simulink model "Top"  (R2020b)
settings: Solver=VariableStepAuto  StartTime=0.0  StopTime=10.0  RelTol=1e-3
libraries: Bibavion x6
settings Model: Creator=Nicolas  LastModifiedBy=Nicolas

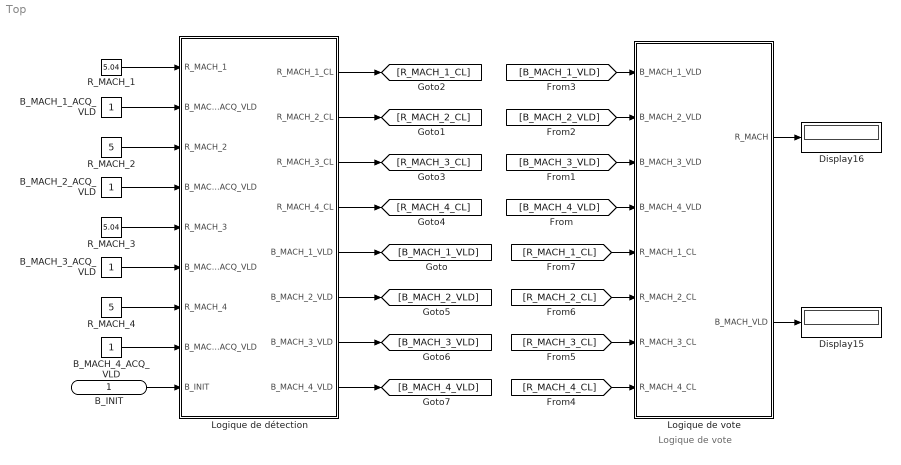
== system Top ==
  note: Logique de vote
  B_INIT : Inport  OutDataTypeStr=boolean
  B_MACH_1_ACQ_VLD : Constant  OutDataTypeStr=boolean
  B_MACH_2_ACQ_VLD : Constant  OutDataTypeStr=boolean
  B_MACH_3_ACQ_VLD : Constant  OutDataTypeStr=boolean
  B_MACH_4_ACQ_VLD : Constant  OutDataTypeStr=boolean
  Display15 : Display
  Display16 : Display
  Logique de détection : Subsystem
  Logique de vote : Subsystem
  R_MACH_1 : Constant  Value=5.04  OutDataTypeStr=single
  R_MACH_2 : Constant  Value=5  OutDataTypeStr=single
  R_MACH_3 : Constant  Value=5.04  OutDataTypeStr=single
  R_MACH_4 : Constant  Value=5  OutDataTypeStr=single
  wires:
  [B_MACH_4_VLD] -> Logique de vote/4(B_MACH_4_VLD)
  [R_MACH_1_CL] -> Logique de vote/5(R_MACH_1_CL)
  Logique de détection/4(R_MACH_4_CL) -> [R_MACH_4_CL]
  R_MACH_1/1 -> Logique de détection/1(R_MACH_1)
  B_MACH_3_ACQ_VLD/1 -> Logique de détection/6(B_MACH_3_ACQ_VLD)
  [R_MACH_4_CL] -> Logique de vote/8(R_MACH_4_CL)
  B_MACH_2_ACQ_VLD/1 -> Logique de détection/4(B_MACH_2_ACQ_VLD)
  Logique de détection/7(B_MACH_3_VLD) -> [B_MACH_3_VLD]
  R_MACH_3/1 -> Logique de détection/5(R_MACH_3)
  [B_MACH_3_VLD] -> Logique de vote/3(B_MACH_3_VLD)
  [R_MACH_3_CL] -> Logique de vote/7(R_MACH_3_CL)
  Logique de vote/2(B_MACH_VLD) -> Display15/1
  [B_MACH_2_VLD] -> Logique de vote/2(B_MACH_2_VLD)
  [R_MACH_2_CL] -> Logique de vote/6(R_MACH_2_CL)
  [B_MACH_1_VLD] -> Logique de vote/1(B_MACH_1_VLD)
  Logique de détection/1(R_MACH_1_CL) -> [R_MACH_1_CL]
  B_MACH_4_ACQ_VLD/1 -> Logique de détection/8(B_MACH_4_ACQ_VLD)
  B_MACH_1_ACQ_VLD/1 -> Logique de détection/2(B_MACH_1_ACQ_VLD)
  R_MACH_2/1 -> Logique de détection/3(R_MACH_2)
  Logique de détection/6(B_MACH_2_VLD) -> [B_MACH_2_VLD]
  Logique de détection/8(B_MACH_4_VLD) -> [B_MACH_4_VLD]
  Logique de détection/5(B_MACH_1_VLD) -> [B_MACH_1_VLD]
  Logique de vote/1(R_MACH) -> Display16/1
  R_MACH_4/1 -> Logique de détection/7(R_MACH_4)
  Logique de détection/2(R_MACH_2_CL) -> [R_MACH_2_CL]
  Logique de détection/3(R_MACH_3_CL) -> [R_MACH_3_CL]
  B_INIT/1 -> Logique de détection/9(B_INIT)

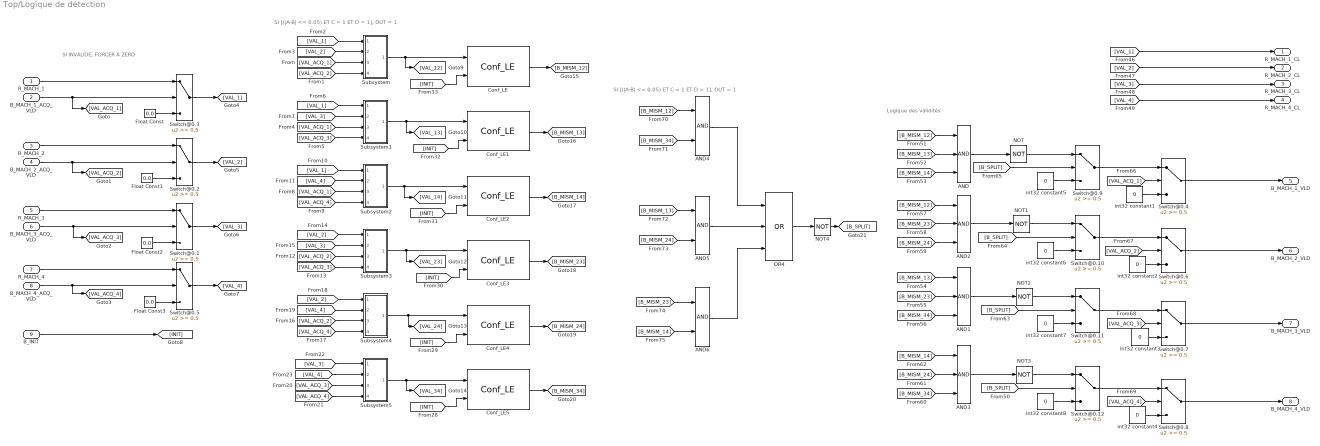
== system Top/Logique de détection ==
  note: SI [(|A-B| <= 0.05) ET C = 1 ET D = 1], OUT = 1
  note: SI INVALIDE, FORCER A ZERO
  note: Logique des validités
  note: SI [(|A-B| <= 0.05) ET C = 1 ET D = 1], OUT = 1
  R_MACH_1 : Inport
  B_MACH_1_ACQ_VLD : Inport  Port=2
  R_MACH_2 : Inport  Port=3
  B_MACH_2_ACQ_VLD : Inport  Port=4
  R_MACH_3 : Inport  Port=5
  B_MACH_3_ACQ_VLD : Inport  Port=6
  R_MACH_4 : Inport  Port=7
  B_MACH_4_ACQ_VLD : Inport  Port=8
  B_INIT : Inport  Port=9
  AND{,1..3} (4 alike) : Logic  Inputs=3  AllPortsSameDT=off  OutDataTypeStr=boolean
  AND4 : Logic  AllPortsSameDT=off  OutDataTypeStr=boolean
  AND5 : Logic  AllPortsSameDT=off  OutDataTypeStr=boolean
  AND6 : Logic  AllPortsSameDT=off  OutDataTypeStr=boolean
  Conf_LE{,1..5} (6 alike) : Bibavion/Logical/Conf_LE  time=2  init=0
      settings: SourceProductName=Bibavion P20
  Float Const{,1..3} (4 alike) : Constant  Value=0.0  OutDataTypeStr=single
  NOT{,1..4} (5 alike) : Logic  Operator=NOT  IconShape=distinctive  AllPortsSameDT=off  OutDataTypeStr=boolean
  OR4 : Logic  Operator=OR  Inputs=3  AllPortsSameDT=off  OutDataTypeStr=boolean
  Subsystem : Subsystem
  Subsystem1 : Subsystem
  Subsystem2 : Subsystem
  Subsystem3 : Subsystem
  Subsystem4 : Subsystem
  Subsystem5 : Subsystem
  Switch@0.{1..12} (12 alike) : Switch  Threshold=0.5
  int32 constant{1..8} (8 alike) : Constant  Value=0  OutDataTypeStr=int32  SampleTime=-1
  R_MACH_1_CL : Outport
  R_MACH_2_CL : Outport  Port=2
  R_MACH_3_CL : Outport  Port=3
  R_MACH_4_CL : Outport  Port=4
  B_MACH_1_VLD : Outport  Port=5
  B_MACH_2_VLD : Outport  Port=6
  B_MACH_3_VLD : Outport  Port=7
  B_MACH_4_VLD : Outport  Port=8
  wires:
  [VAL_ACQ_2] -> Subsystem4/3(In3)
  Float Const3/1 -> Switch@0.5/3
  [VAL_ACQ_2] -> Subsystem/4(In4)
  B_MACH_3_ACQ_VLD/1 -> [VAL_ACQ_3], Switch@0.1/2
  NOT1/1 -> Switch@0.10/1
  [B_MISM_23] -> AND1/2
  [VAL_ACQ_1] -> Subsystem2/3(In3)
  Switch@0.11/1 -> Switch@0.7/1
  AND4/1 -> OR4/1
  [VAL_4] -> Subsystem4/2(In2)
  [B_MISM_24] -> AND2/3
  Switch@0.3/1 -> [VAL_1]
  B_MACH_4_ACQ_VLD/1 -> Switch@0.5/2, [VAL_ACQ_4]
  B_MACH_1_ACQ_VLD/1 -> [VAL_ACQ_1], Switch@0.3/2
  Subsystem1/1(Out1) -> [VAL_13], Conf_LE1/1
  Switch@0.12/1 -> Switch@0.8/1
  [VAL_3] -> Subsystem1/2(In2)
  [VAL_ACQ_3] -> Subsystem1/4(In4)
  Float Const1/1 -> Switch@0.2/3
  [VAL_ACQ_1] -> Subsystem/3(In3)
  [VAL_1] -> Subsystem1/1(In1)
  Conf_LE3/1 -> [B_MISM_23]
  [VAL_2] -> Subsystem4/1(In1)
  [INIT] -> Conf_LE5/2
  Switch@0.2/1 -> [VAL_2]
  Conf_LE1/1 -> [B_MISM_13]
  Switch@0.8/1 -> B_MACH_4_VLD/1
  Subsystem5/1(Out1) -> [VAL_34], Conf_LE5/1
  B_MACH_2_ACQ_VLD/1 -> [VAL_ACQ_2], Switch@0.2/2
  [VAL_3] -> Subsystem3/2(In2)
  Switch@0.1/1 -> [VAL_3]
  [B_MISM_14] -> AND3/1
  [VAL_2] -> Subsystem3/1(In1)
  [VAL_2] -> Subsystem/2(In2)
  [VAL_ACQ_3] -> Switch@0.7/2
  Subsystem4/1(Out1) -> [VAL_24], Conf_LE4/1
  [VAL_1] -> R_MACH_1_CL/1
  [VAL_4] -> Subsystem2/2(In2)
  int32 constant3/1 -> Switch@0.7/3
  NOT4/1 -> [B_SPLIT]
  [VAL_4] -> Subsystem5/2(In2)
  Switch@0.7/1 -> B_MACH_3_VLD/1
  [VAL_ACQ_3] -> Subsystem5/3(In3)
  AND/1 -> NOT/1
  [VAL_ACQ_3] -> Subsystem3/4(In4)
  [B_MISM_24] -> AND5/2
  AND3/1 -> NOT3/1
  Subsystem2/1(Out1) -> [VAL_14], Conf_LE2/1
  [INIT] -> Conf_LE4/2
  [B_SPLIT] -> Switch@0.11/2
  [VAL_ACQ_4] -> Subsystem2/4(In4)
  R_MACH_1/1 -> Switch@0.3/1
  [INIT] -> Conf_LE2/2
  [VAL_ACQ_2] -> Subsystem3/3(In3)
  Float Const2/1 -> Switch@0.1/3
  Float Const/1 -> Switch@0.3/3
  [VAL_ACQ_4] -> Subsystem4/4(In4)
  [VAL_ACQ_2] -> Switch@0.6/2
  Subsystem/1(Out1) -> [VAL_12], Conf_LE/1
  Subsystem3/1(Out1) -> [VAL_23], Conf_LE3/1
  [VAL_1] -> Subsystem/1(In1)
  [VAL_2] -> R_MACH_2_CL/1
  Switch@0.10/1 -> Switch@0.6/1
  [INIT] -> Conf_LE/2
  [VAL_4] -> R_MACH_4_CL/1
  [VAL_ACQ_4] -> Subsystem5/4(In4)
  [B_MISM_13] -> AND5/1
  Switch@0.5/1 -> [VAL_4]
  AND6/1 -> OR4/3
  [VAL_1] -> Subsystem2/1(In1)
  [VAL_ACQ_1] -> Subsystem1/3(In3)
  NOT2/1 -> Switch@0.11/1
  [INIT] -> Conf_LE3/2
  [INIT] -> Conf_LE1/2
  [VAL_3] -> Subsystem5/1(In1)
  Conf_LE4/1 -> [B_MISM_24]
  int32 constant4/1 -> Switch@0.8/3
  [B_MISM_23] -> AND6/1
  Conf_LE/1 -> [B_MISM_12]
  [VAL_ACQ_4] -> Switch@0.8/2
  AND1/1 -> NOT2/1
  AND2/1 -> NOT1/1
  Conf_LE2/1 -> [B_MISM_14]
  [VAL_ACQ_1] -> Switch@0.4/2
  [B_MISM_14] -> AND/3
  [B_MISM_13] -> AND/2
  NOT/1 -> Switch@0.9/1
  [B_MISM_12] -> AND4/1
  [B_MISM_34] -> AND3/3
  Conf_LE5/1 -> [B_MISM_34]
  AND5/1 -> OR4/2
  int32 constant6/1 -> Switch@0.10/3
  [B_SPLIT] -> Switch@0.10/2
  int32 constant2/1 -> Switch@0.6/3
  [B_MISM_13] -> AND1/1
  [B_MISM_12] -> AND2/1
  [B_MISM_23] -> AND2/2
  Switch@0.4/1 -> B_MACH_1_VLD/1
  [B_MISM_12] -> AND/1
  OR4/1 -> NOT4/1
  int32 constant8/1 -> Switch@0.12/3
  [B_MISM_34] -> AND1/3
  [B_SPLIT] -> Switch@0.9/2
  [B_MISM_24] -> AND3/2
  NOT3/1 -> Switch@0.12/1
  int32 constant1/1 -> Switch@0.4/3
  [VAL_3] -> R_MACH_3_CL/1
  [B_MISM_14] -> AND6/2
  [B_MISM_34] -> AND4/2
  Switch@0.6/1 -> B_MACH_2_VLD/1
  int32 constant7/1 -> Switch@0.11/3
  Switch@0.9/1 -> Switch@0.4/1
  [B_SPLIT] -> Switch@0.12/2
  int32 constant5/1 -> Switch@0.9/3
  B_INIT/1 -> [INIT]
  R_MACH_2/1 -> Switch@0.2/1
  R_MACH_4/1 -> Switch@0.5/1
  R_MACH_3/1 -> Switch@0.1/1

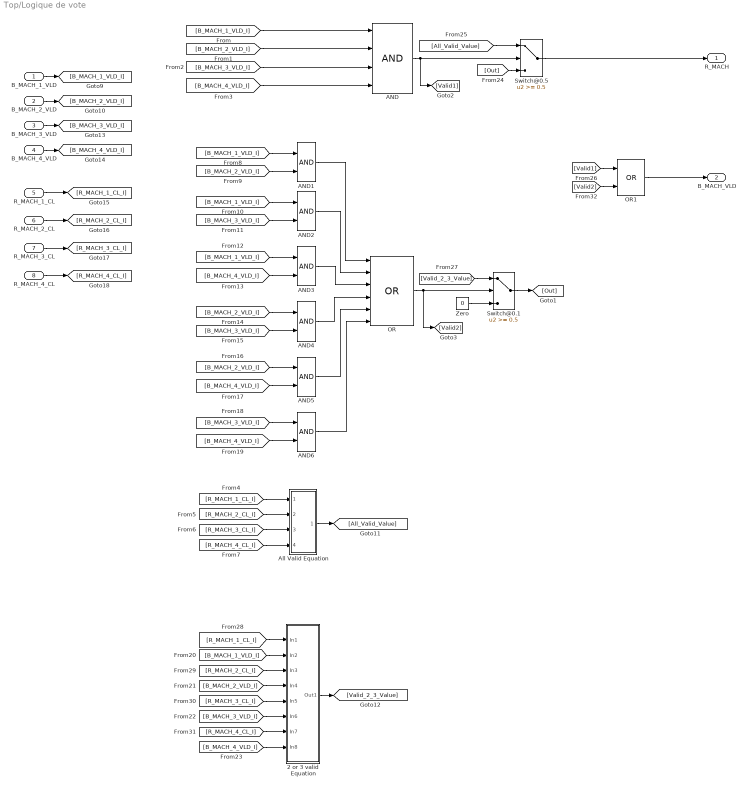
== system Top/Logique de vote ==
  B_MACH_1_VLD : Inport
  B_MACH_2_VLD : Inport  Port=2
  B_MACH_3_VLD : Inport  Port=3
  B_MACH_4_VLD : Inport  Port=4
  R_MACH_1_CL : Inport  Port=5
  R_MACH_2_CL : Inport  Port=6
  R_MACH_3_CL : Inport  Port=7
  R_MACH_4_CL : Inport  Port=8
  2 or 3 valid Equation : Subsystem
  AND : Logic  Inputs=4  IconShape=distinctive  AllPortsSameDT=off  OutDataTypeStr=boolean
  AND{1..6} (6 alike) : Logic  IconShape=distinctive  AllPortsSameDT=off  OutDataTypeStr=boolean
  All Valid Equation : Subsystem
  OR : Logic  Operator=OR  Inputs=6  IconShape=distinctive  AllPortsSameDT=off  OutDataTypeStr=boolean
  OR1 : Logic  Operator=OR  IconShape=distinctive  AllPortsSameDT=off  OutDataTypeStr=boolean
  Switch@0.1 : Switch  Threshold=0.5
  Switch@0.5 : Switch  Threshold=0.5
  Zero : Constant  Value=0  OutDataTypeStr=single
  R_MACH : Outport
  B_MACH_VLD : Outport  Port=2
  wires:
  [B_MACH_2_VLD_I] -> AND1/2
  B_MACH_3_VLD/1 -> [B_MACH_3_VLD_I]
  [B_MACH_2_VLD_I] -> AND/2
  [B_MACH_4_VLD_I] -> AND/4
  [B_MACH_1_VLD_I] -> AND/1
  R_MACH_2_CL/1 -> [R_MACH_2_CL_I]
  [B_MACH_3_VLD_I] -> AND2/2
  R_MACH_1_CL/1 -> [R_MACH_1_CL_I]
  [R_MACH_2_CL_I] -> All Valid Equation/2(In2)
  [B_MACH_4_VLD_I] -> AND3/2
  AND2/1 -> OR/2
  [B_MACH_2_VLD_I] -> AND5/1
  [B_MACH_1_VLD_I] -> AND2/1
  [B_MACH_3_VLD_I] -> AND4/2
  [B_MACH_3_VLD_I] -> AND/3
  R_MACH_4_CL/1 -> [R_MACH_4_CL_I]
  AND4/1 -> OR/4
  B_MACH_1_VLD/1 -> [B_MACH_1_VLD_I]
  AND/1 -> [Valid1], Switch@0.5/2
  [R_MACH_4_CL_I] -> 2 or 3 valid Equation/7(In7)
  [B_MACH_3_VLD_I] -> AND6/1
  [Valid_2_3_Value] -> Switch@0.1/1
  AND5/1 -> OR/5
  OR/1 -> [Valid2], Switch@0.1/2
  [B_MACH_1_VLD_I] -> AND1/1
  [B_MACH_1_VLD_I] -> AND3/1
  [B_MACH_3_VLD_I] -> 2 or 3 valid Equation/6(In6)
  B_MACH_4_VLD/1 -> [B_MACH_4_VLD_I]
  [B_MACH_4_VLD_I] -> AND6/2
  [R_MACH_1_CL_I] -> All Valid Equation/1(In1)
  2 or 3 valid Equation/1(Out1) -> [Valid_2_3_Value]
  [R_MACH_3_CL_I] -> All Valid Equation/3(In3)
  [B_MACH_4_VLD_I] -> AND5/2
  [B_MACH_1_VLD_I] -> 2 or 3 valid Equation/2(In2)
  [R_MACH_3_CL_I] -> 2 or 3 valid Equation/5(In5)
  [R_MACH_4_CL_I] -> All Valid Equation/4(In4)
  All Valid Equation/1(Out1) -> [All_Valid_Value]
  [All_Valid_Value] -> Switch@0.5/1
  AND3/1 -> OR/3
  [R_MACH_1_CL_I] -> 2 or 3 valid Equation/1(In1)
  [B_MACH_2_VLD_I] -> 2 or 3 valid Equation/4(In4)
  [R_MACH_2_CL_I] -> 2 or 3 valid Equation/3(In3)
  AND6/1 -> OR/6
  [B_MACH_4_VLD_I] -> 2 or 3 valid Equation/8(In8)
  [B_MACH_2_VLD_I] -> AND4/1
  AND1/1 -> OR/1
  Zero/1 -> Switch@0.1/3
  R_MACH_3_CL/1 -> [R_MACH_3_CL_I]
  Switch@0.5/1 -> R_MACH/1
  B_MACH_2_VLD/1 -> [B_MACH_2_VLD_I]
  Switch@0.1/1 -> [Out]
  [Out] -> Switch@0.5/3
  [Valid1] -> OR1/1
  [Valid2] -> OR1/2
  OR1/1 -> B_MACH_VLD/1

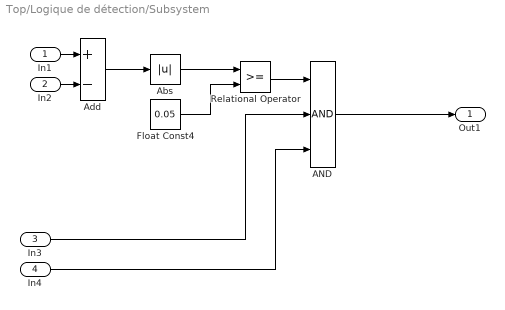
== system Top/Logique de détection/Subsystem ==
  In1 : Inport
  In2 : Inport  Port=2
  In3 : Inport  Port=3
  In4 : Inport  Port=4
  AND : Logic  Inputs=3  AllPortsSameDT=off  OutDataTypeStr=boolean
  Abs : Abs
  Add : Sum  Inputs=+-
  Float Const4 : Constant  Value=0.05  OutDataTypeStr=single
  Relational Operator : RelationalOperator  OutDataTypeStr=boolean  RndMeth=Nearest
  Out1 : Outport
  wires:
  In3/1 -> AND/2
  In4/1 -> AND/3
  Add/1 -> Abs/1
  Relational Operator/1 -> AND/1
  Abs/1 -> Relational Operator/1
  AND/1 -> Out1/1
  Float Const4/1 -> Relational Operator/2
  In2/1 -> Add/2
  In1/1 -> Add/1

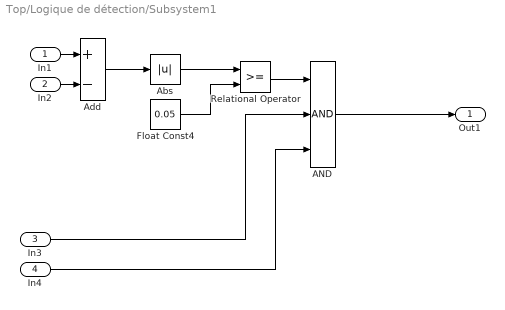
== system Top/Logique de détection/Subsystem1 ==
  In1 : Inport
  In2 : Inport  Port=2
  In3 : Inport  Port=3
  In4 : Inport  Port=4
  AND : Logic  Inputs=3  AllPortsSameDT=off  OutDataTypeStr=boolean
  Abs : Abs
  Add : Sum  Inputs=+-
  Float Const4 : Constant  Value=0.05  OutDataTypeStr=single
  Relational Operator : RelationalOperator  OutDataTypeStr=boolean  RndMeth=Nearest
  Out1 : Outport
  wires:
  In3/1 -> AND/2
  In4/1 -> AND/3
  Add/1 -> Abs/1
  Relational Operator/1 -> AND/1
  Abs/1 -> Relational Operator/1
  AND/1 -> Out1/1
  Float Const4/1 -> Relational Operator/2
  In2/1 -> Add/2
  In1/1 -> Add/1

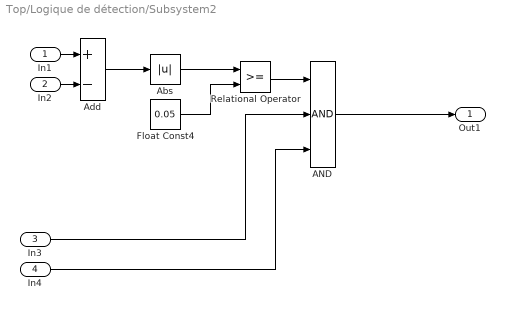
== system Top/Logique de détection/Subsystem2 ==
  In1 : Inport
  In2 : Inport  Port=2
  In3 : Inport  Port=3
  In4 : Inport  Port=4
  AND : Logic  Inputs=3  AllPortsSameDT=off  OutDataTypeStr=boolean
  Abs : Abs
  Add : Sum  Inputs=+-
  Float Const4 : Constant  Value=0.05  OutDataTypeStr=single
  Relational Operator : RelationalOperator  OutDataTypeStr=boolean  RndMeth=Nearest
  Out1 : Outport
  wires:
  In3/1 -> AND/2
  In4/1 -> AND/3
  Add/1 -> Abs/1
  Relational Operator/1 -> AND/1
  Abs/1 -> Relational Operator/1
  AND/1 -> Out1/1
  Float Const4/1 -> Relational Operator/2
  In2/1 -> Add/2
  In1/1 -> Add/1

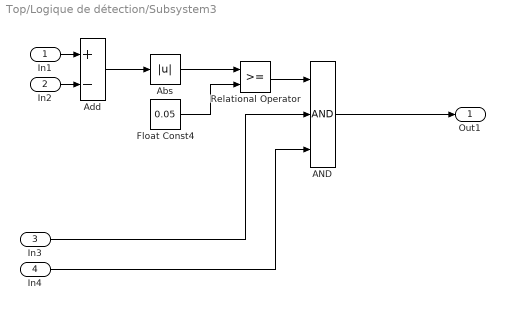
== system Top/Logique de détection/Subsystem3 ==
  In1 : Inport
  In2 : Inport  Port=2
  In3 : Inport  Port=3
  In4 : Inport  Port=4
  AND : Logic  Inputs=3  AllPortsSameDT=off  OutDataTypeStr=boolean
  Abs : Abs
  Add : Sum  Inputs=+-
  Float Const4 : Constant  Value=0.05  OutDataTypeStr=single
  Relational Operator : RelationalOperator  OutDataTypeStr=boolean  RndMeth=Nearest
  Out1 : Outport
  wires:
  In3/1 -> AND/2
  In4/1 -> AND/3
  Add/1 -> Abs/1
  Relational Operator/1 -> AND/1
  Abs/1 -> Relational Operator/1
  AND/1 -> Out1/1
  Float Const4/1 -> Relational Operator/2
  In2/1 -> Add/2
  In1/1 -> Add/1

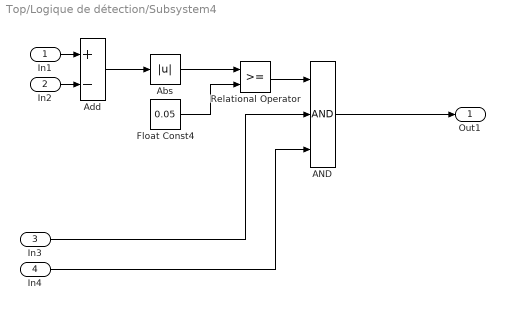
== system Top/Logique de détection/Subsystem4 ==
  In1 : Inport
  In2 : Inport  Port=2
  In3 : Inport  Port=3
  In4 : Inport  Port=4
  AND : Logic  Inputs=3  AllPortsSameDT=off  OutDataTypeStr=boolean
  Abs : Abs
  Add : Sum  Inputs=+-
  Float Const4 : Constant  Value=0.05  OutDataTypeStr=single
  Relational Operator : RelationalOperator  OutDataTypeStr=boolean  RndMeth=Nearest
  Out1 : Outport
  wires:
  In3/1 -> AND/2
  In4/1 -> AND/3
  Add/1 -> Abs/1
  Relational Operator/1 -> AND/1
  Abs/1 -> Relational Operator/1
  AND/1 -> Out1/1
  Float Const4/1 -> Relational Operator/2
  In2/1 -> Add/2
  In1/1 -> Add/1

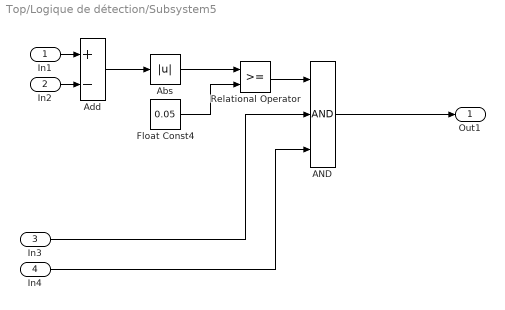
== system Top/Logique de détection/Subsystem5 ==
  In1 : Inport
  In2 : Inport  Port=2
  In3 : Inport  Port=3
  In4 : Inport  Port=4
  AND : Logic  Inputs=3  AllPortsSameDT=off  OutDataTypeStr=boolean
  Abs : Abs
  Add : Sum  Inputs=+-
  Float Const4 : Constant  Value=0.05  OutDataTypeStr=single
  Relational Operator : RelationalOperator  OutDataTypeStr=boolean  RndMeth=Nearest
  Out1 : Outport
  wires:
  In3/1 -> AND/2
  In4/1 -> AND/3
  Add/1 -> Abs/1
  Relational Operator/1 -> AND/1
  Abs/1 -> Relational Operator/1
  AND/1 -> Out1/1
  Float Const4/1 -> Relational Operator/2
  In2/1 -> Add/2
  In1/1 -> Add/1

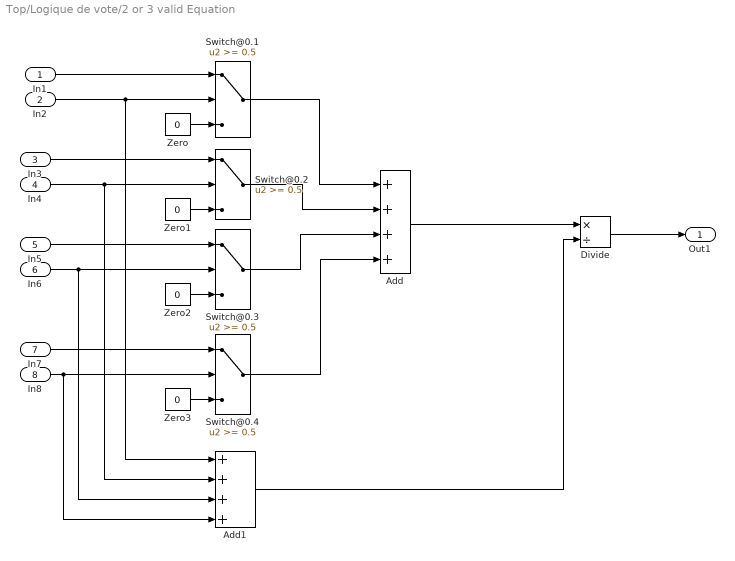
== system Top/Logique de vote/2 or 3 valid Equation ==
  In1 : Inport
  In2 : Inport  Port=2
  In3 : Inport  Port=3
  In4 : Inport  Port=4
  In5 : Inport  Port=5
  In6 : Inport  Port=6
  In7 : Inport  Port=7
  In8 : Inport  Port=8
  Add : Sum  Inputs=++++
  Add1 : Sum  Inputs=++++
  Divide : Product  Inputs=*/
  Switch@0.{1..4} (4 alike) : Switch  Threshold=0.5
  Zero{,1..3} (4 alike) : Constant  Value=0  OutDataTypeStr=single
  Out1 : Outport
  wires:
  Add/1 -> Divide/1
  Zero3/1 -> Switch@0.4/3
  Zero/1 -> Switch@0.1/3
  Switch@0.3/1 -> Add/3
  Divide/1 -> Out1/1
  Switch@0.4/1 -> Add/4
  Zero2/1 -> Switch@0.3/3
  Zero1/1 -> Switch@0.2/3
  In1/1 -> Switch@0.1/1
  In5/1 -> Switch@0.3/1
  Switch@0.1/1 -> Add/1
  Switch@0.2/1 -> Add/2
  In3/1 -> Switch@0.2/1
  In2/1 -> Add1/1, Switch@0.1/2
  In6/1 -> Add1/3, Switch@0.3/2
  In8/1 -> Add1/4, Switch@0.4/2
  In4/1 -> Add1/2, Switch@0.2/2
  In7/1 -> Switch@0.4/1
  Add1/1 -> Divide/2

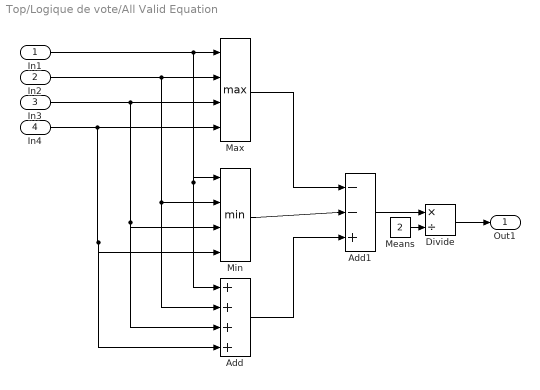
== system Top/Logique de vote/All Valid Equation ==
  In1 : Inport
  In2 : Inport  Port=2
  In3 : Inport  Port=3
  In4 : Inport  Port=4
  Add : Sum  Inputs=++++
  Add1 : Sum  Inputs=--+
  Divide : Product  Inputs=*/
  Max : MinMax  Function=max  Inputs=4
  Means : Constant  Value=2  OutDataTypeStr=single
  Min : MinMax  Inputs=4
  Out1 : Outport
  wires:
  Add1/1 -> Divide/1
  In2/1 -> Add/2, Min/2, Max/2
  In3/1 -> Add/3, Min/3, Max/3
  Divide/1 -> Out1/1
  Means/1 -> Divide/2
  In1/1 -> Min/1, Add/1, Max/1
  In4/1 -> Add/4, Min/4, Max/4
  Max/1 -> Add1/1
  Min/1 -> Add1/2
  Add/1 -> Add1/3
